simulink model "ProblemF_xm_t2"  (R2018b)
settings: Solver=VariableStepAuto  StartTime=0.0  StopTime=10.0  RelTol=1e-3
undefined symbols (not defined in the file): A, B, C
libraries: peLuenbergerObserver x1
settings Model: Creator=Pranali  LastModifiedBy=Pranali

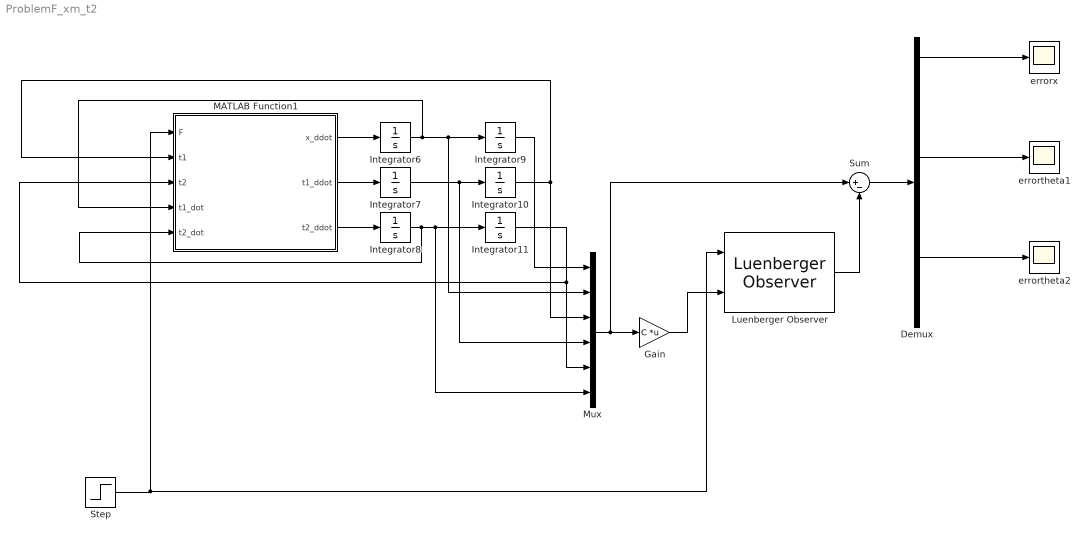
== system ProblemF_xm_t2 ==
  Demux : Demux  Outputs=6
  Gain : Gain  Gain=C  Multiplication=Matrix(K*u)
  Integrator{6..11} (6 alike) : Integrator
  "Luenberger Observer " : peLuenbergerObserver/Luenberger Observer  StateSpaceType=Continuous-time  Ad=A  Bd=B  Cd=C  Dd=D  A=A  B=B  C=C  D=[0;0]  ObserverDesign=Observer gain  Ld=L  DesiredEigenvalues=[-0.2 -0.3 -0.4 -0.5 -0.6 -0.7]  x0="[1 0  pi/6 0  pi/6 0]"  Tsd=0.1  Ts=0.1
  MATLAB Function1 : MATLAB Function  TreatAsAtomicUnit=on
  Mux : Mux  Inputs=6
  Step : Step  Time=10  SampleTime=0
  Sum : Sum  Inputs=|+-
  errortheta1 : Scope
  errortheta2 : Scope
  errorx : Scope
  wires:
  Gain/1 -> "Luenberger Observer "/2
  Demux/5 -> errortheta2/1
  Step/1 -> "Luenberger Observer "/1, MATLAB Function1/1(F)
  Integrator6/1 -> MATLAB Function1/4(t1_dot), Mux/2, Integrator9/1
  Integrator10/1 -> MATLAB Function1/2(t1), Mux/3
  MATLAB Function1/3(t2_ddot) -> Integrator8/1
  Sum/1 -> Demux/1
  Integrator8/1 -> MATLAB Function1/5(t2_dot), Mux/6, Integrator11/1
  MATLAB Function1/1(x_ddot) -> Integrator6/1
  Integrator9/1 -> Mux/1
  Integrator7/1 -> Mux/4, Integrator10/1
  Integrator11/1 -> Mux/5, MATLAB Function1/3(t2)
  "Luenberger Observer "/1 -> Sum/2
  Demux/1 -> errorx/1
  MATLAB Function1/2(t1_ddot) -> Integrator7/1
  Mux/1 -> Sum/1, Gain/1
  Demux/3 -> errortheta1/1

== matlab function ProblemF_xm_t2/MATLAB Function1 ==
  data: F input; t1 input; t2 input; x_ddot output; t1_dot input; t2_dot input; t1_ddot output; t2_ddot output
function [x_ddot,t1_ddot,t2_ddot] = NonLinear_Simulationluenberger(F,t1,t2,t1_dot,t2_dot)

%% System Parameters
l1 = 20; % length l1
l2 = 10; % length l2
m1 = 100; % mass m1
m2 = 100; % mass m2
M = 1000; % mass M
g = 9.8; % acceleration due to gravity

%% Trignometric Variables
c1 = cos(t1);
c2 = cos(t2);
s1 = sin(t1);
s2 = sin(t2);

%% x_ddot equation 
x_ddot = (F - m1*c1*s1*g - m2*c2*s2*g - m1*l1*(t1_dot^2)*(s1) - m2*l2*(t2_dot^2)*(s2))/(M + m1*(s1^2) + m2*(s2^2));

%% t1_ddot equation
t1_ddot = (x_ddot*c1 - g*s1)/l1;

%% t2_ddot equation
t2_ddot = (x_ddot*c2 - g*s2)/l2;

end
